simulink model "ROPOD_Control_SIM"  (R2017b)
settings: Solver=VariableStepAuto  StartTime=0.0  StopTime=inf  RelTol=1e-3
values from neighbouring files (symbols this model uses):
  AgentNumber = 1    [init_model.m]
  FFtheta_intia = 0    [init_model.m]
  FFxy_mass = 0*80    (= 0)    [init_model.m]
  flock_FFtheta_friction = 50    [init_model.m]
  flock_FFxy_friction = 100    [init_model.m]
  I_fhz_ddelta_cntr = 0    [init_model.m]
  I_fhz_dtheta_cntr = 0.3    [init_model.m]
  I_fhz_dtheta_flock_cntr = 0.1    [init_model.m]
  I_fhz_dvarphi_cntr = 0    [init_model.m]
  I_fhz_dxdy_cntr = 0.25    [init_model.m]
  I_fhz_dxdy_flock_cntr = 0.1    [init_model.m]
  K_gain_ddelta_cntr = 0.1    [init_model.m]
  K_gain_dtheta_cntr = 150    [init_model.m]
  K_gain_dtheta_flock_cntr = 100    [init_model.m]
  K_gain_dvarphi_cntr = 0.05    [init_model.m]
  K_gain_dxdy_cntr = 200    [init_model.m]
  K_gain_dxdy_flock_cntr = 200    [init_model.m]
  LL_wp_fhz_ddelta_cntr = 2    [init_model.m]
  LL_wp_fhz_dtheta_cntr = 20    [init_model.m]
  LL_wp_fhz_dtheta_flock_cntr = 20    [init_model.m]
  LL_wp_fhz_dvarphi_cntr = 10    [init_model.m]
  LL_wp_fhz_dxdy_cntr = 20    [init_model.m]
  LL_wp_fhz_dxdy_flock_cntr = 20    [init_model.m]
  LL_wz_fhz_ddelta_cntr = 2    [init_model.m]
  LL_wz_fhz_dtheta_cntr = 20    [init_model.m]
  LL_wz_fhz_dtheta_flock_cntr = 20    [init_model.m]
  LL_wz_fhz_dvarphi_cntr = 2    [init_model.m]
  LL_wz_fhz_dxdy_cntr = 20    [init_model.m]
  LL_wz_fhz_dxdy_flock_cntr = 20    [init_model.m]
  LPF_fhz_ddelta_cntr = 50    [init_model.m]
  LPF_fhz_ddelta_meas = 50    [init_model.m]
  LPF_fhz_dtheta_cntr = 100    [init_model.m]
  LPF_fhz_dtheta_flock_cntr = 40    [init_model.m]
  LPF_fhz_dvarphi_cntr = 50    [init_model.m]
  LPF_fhz_dvarphi_meas = 50    [init_model.m]
  LPF_fhz_dxdy_cntr = 100    [init_model.m]
  LPF_fhz_dxdy_flock_cntr = 40    [init_model.m]
  max_flock_acc_theta = 0.5    [init_model.m]
  max_flock_acc_xy = 0.5    [init_model.m]
  max_flock_vel_theta = 1.0    (= 1)    [init_model.m]
  max_flock_vel_xy = 1.0    (= 1)    [init_model.m]
  max_hw_tau = 7.0    (= 7)    [init_model.m]
  max_ropod_acc_theta = 1.6    [init_model.m]
  max_ropod_acc_xy = 2.0    (= 2)    [init_model.m]
  max_ropod_sw_force = 500    [init_model.m]
  max_ropod_sw_tau = 250    [init_model.m]
  max_ropod_vel_theta = 1.6    [init_model.m]
  max_ropod_vel_xy = 2.0    (= 2)    [init_model.m]
  max_sw_current = 10    [init_model.m]
  Nagents = 2    [init_model.m]
  Nwheels = 4    [Jqwl_numeric_function.m]    (also in S_matrix.m; extract_kinmodel_parameters.m; init_model.m; tau_optimal_dist_vec_fun.m)
  pivot_offs_sws = [0.0243    0.4689    0.3384    5.9050]    [init_model.m]
  ropod_kinmodel_pv = struct2array(ropod_kinmodel_param)    [set_ropod_KinModparams.m]
  ropod_position_inflock = [-1 0 3.1416]    [init_model.m]
  SW_COM1_ENABLE1 = hex2dec('0001')    [init_model.m]
  SW_COM1_ENABLE2 = hex2dec('0002')    [init_model.m]
  SW_COM1_MODE_TORQUE = bitshift(hex2dec('0000'),2)    [init_model.m]
  SW_COM1_MODE_VELOCITY = bitshift(hex2dec('0002'),2)    [init_model.m]
  SW_COM1_USE_TS = hex2dec('8000')    [init_model.m]
  sw_tau_2_current = 1/motor_physical_parameters.torqueconstant.value    [init_model.m]
  Tinit = 2    [init_model.m]
  Ts = 0.001    [init_model.m]
  Ts_MPC = 0.01    [init_model.m]
  Tsflck = 0.01    [init_model.m]
undefined symbols (not defined in the file or in its folder): acc_limit, accmax, b_cx, b_cy, b_rx, bus_size, comp_enable, Desired, DiscIntNeverNeededParam, Fcgain, gdis, k_cx, k_cy, live_tuning, m_robot, Nominal, Nominal_x, Nominal_y, offsets, portwidth, sizes, types, vel_limit, vmax1, vmax2
libraries: simulink x90, cstblocks x66, dspsigops x12, dspnetwork x4
(part 8 of 8)

== matlab function ROPOD_Control_SIM/RopodTorqueDistribution/wheel flip compensation/MATLAB Function2 ==
  data: tl input; tl_out output; tr input; ropod_kinmodel_param_vec input size=18; tr_out output; kmax input; sc output; Fthr input; tau_max input
function [tl_out,tr_out, sc] = fcn(tl, tr, ropod_kinmodel_param_vec, kmax, Fthr, tau_max)

[  rW1_1,rW1_2,rW1_3,rW1_4,rW2_1,rW2_2,rW2_3,rW2_4,...
    s_w,...
    d_w, ...
    CW1_1,CW1_2,CW1_3,CW1_4,CW2_1,CW2_2,CW2_3,CW2_4 ...
    ]= extract_kinmodel_parameters(ropod_kinmodel_param_vec);

Fxi = (tl/rW1_1+tr/rW1_2);
Fyi = (tr/rW1_2-tl/rW1_1)*(d_w/(2*s_w));
theta = atan2(Fyi,Fxi);

Fsize = abs(Fyi);
if Fsize> Fthr
   sc = (1+(kmax-1)*abs( sin(theta)) );
else
    sc = 1;
end

avg_t = (tr+tl)/2;
diff_t = (tr-tl)/2;
tl_out = avg_t-sc*diff_t;
tr_out = avg_t+sc*diff_t;

if(abs(tl_out)>tau_max && abs(tl_out)>abs(tr_out))
    sc = tau_max/abs(tl_out);
    tl_out = sc*tl_out;
    tr_out = sc*tr_out;
end

if(abs(tr_out)>tau_max && abs(tr_out)>abs(tl_out))
    sc = tau_max/abs(tr_out);
    tl_out = sc*tl_out;
    tr_out = sc*tr_out;
end

== matlab function ROPOD_Control_SIM/RopodTorqueDistribution/wheel flip compensation/MATLAB Function3 ==
  data: tl input; tl_out output; tr input; ropod_kinmodel_param_vec input size=18; tr_out output; kmax input; sc output; Fthr input; tau_max input
function [tl_out,tr_out, sc] = fcn(tl, tr, ropod_kinmodel_param_vec, kmax, Fthr, tau_max)

[  rW1_1,rW1_2,rW1_3,rW1_4,rW2_1,rW2_2,rW2_3,rW2_4,...
    s_w,...
    d_w, ...
    CW1_1,CW1_2,CW1_3,CW1_4,CW2_1,CW2_2,CW2_3,CW2_4 ...
    ]= extract_kinmodel_parameters(ropod_kinmodel_param_vec);

Fxi = (tl/rW1_1+tr/rW1_2);
Fyi = (tr/rW1_2-tl/rW1_1)*(d_w/(2*s_w));
theta = atan2(Fyi,Fxi);

Fsize = abs(Fyi);
if Fsize> Fthr
   sc = (1+(kmax-1)*abs( sin(theta)) );
else
    sc = 1;
end

avg_t = (tr+tl)/2;
diff_t = (tr-tl)/2;
tl_out = avg_t-sc*diff_t;
tr_out = avg_t+sc*diff_t;

if(abs(tl_out)>tau_max && abs(tl_out)>abs(tr_out))
    sc = tau_max/abs(tl_out);
    tl_out = sc*tl_out;
    tr_out = sc*tr_out;
end

if(abs(tr_out)>tau_max && abs(tr_out)>abs(tl_out))
    sc = tau_max/abs(tr_out);
    tl_out = sc*tl_out;
    tr_out = sc*tr_out;
end

== matlab function ROPOD_Control_SIM/RopodTorqueDistribution/Torque distribution using pseudoinverse/platform_forces_2_tau_dist_optimal_pseudo_inverse ==
  data: GtSl input; taubody input; ena_w input; varphi_tau output; tau_max input; taubody_sc output
function [varphi_tau, taubody_sc]   = Ttaud_optimal_vec( GtSl, taubody, ena_w , tau_max)
%#codegen

Nwheels = 4;

% Optimization
M = eye(2*Nwheels);
for idx = 1:Nwheels
    M(2*(idx-1)+1,2*(idx-1)+1) = ena_w(idx);
    M(2*(idx-1)+2,2*(idx-1)+2) = ena_w(idx);
end
GtM = GtSl*M;

varphi_tau_int = pinv(GtM)*taubody;
varphi_tau_int_max = max(abs(varphi_tau_int));
 

if(varphi_tau_int_max > tau_max)
    taubody_sc = tau_max/varphi_tau_int_max;
else
    taubody_sc = 1.0;
end

varphi_tau = taubody_sc*varphi_tau_int;

end

== matlab function ROPOD_Control_SIM/FlockController/MATLAB Function ==
  data: w_agents_setp input; agents_setp output; d_agents_setp input
function agents_setp = fcn(w_agents_setp, d_agents_setp)

% 3 from three degrees of freedom
% 2 from 1 wrench command +1 velocity command
Nagents = (length(w_agents_setp)/3)+1;
agents_setp_ = zeros(1,2*3*(Nagents-1));

for i_agnt = 1:Nagents-1
    agents_setp_(2*3*(i_agnt-1)+1:2*3*(i_agnt-1)+3) = w_agents_setp(3*(i_agnt-1)+1:3*(i_agnt-1)+3);
    agents_setp_(2*3*(i_agnt-1)+4:2*3*(i_agnt-1)+6) = d_agents_setp(3*(i_agnt-1)+1:3*(i_agnt-1)+3);
end

agents_setp = agents_setp_;

== matlab function ROPOD_Control_SIM/RopodTorqueDistribution/wheel flip compensation/MATLAB Function4 ==
  data: tl input; tl_out output; tr input; ropod_kinmodel_param_vec input size=18; tr_out output; kmax input; sc output; Fthr input; tau_max input
function [tl_out,tr_out, sc] = fcn(tl, tr, ropod_kinmodel_param_vec, kmax, Fthr, tau_max)

[  rW1_1,rW1_2,rW1_3,rW1_4,rW2_1,rW2_2,rW2_3,rW2_4,...
    s_w,...
    d_w, ...
    CW1_1,CW1_2,CW1_3,CW1_4,CW2_1,CW2_2,CW2_3,CW2_4 ...
    ]= extract_kinmodel_parameters(ropod_kinmodel_param_vec);

Fxi = (tl/rW1_1+tr/rW1_2);
Fyi = (tr/rW1_2-tl/rW1_1)*(d_w/(2*s_w));
theta = atan2(Fyi,Fxi);

Fsize = abs(Fyi);
if Fsize> Fthr
   sc = (1+(kmax-1)*abs( sin(theta)) );
else
    sc = 1;
end

avg_t = (tr+tl)/2;
diff_t = (tr-tl)/2;
tl_out = avg_t-sc*diff_t;
tr_out = avg_t+sc*diff_t;

if(abs(tl_out)>tau_max && abs(tl_out)>abs(tr_out))
    sc = tau_max/abs(tl_out);
    tl_out = sc*tl_out;
    tr_out = sc*tr_out;
end

if(abs(tr_out)>tau_max && abs(tr_out)>abs(tl_out))
    sc = tau_max/abs(tr_out);
    tl_out = sc*tl_out;
    tr_out = sc*tr_out;
end

== matlab function ROPOD_Control_SIM/RopodProcessWheelSensorData/Odometry and Measurement model 4SW/Jqwl_numeric ==
  data: ropod_kinmodel_param_vec input; v output; delta input; dvarphi input; ena_w input
function v = Jqwl_numeric_wrapper(ropod_kinmodel_param_vec,  delta, dvarphi, ena_w)

v = Jqwl_numeric_function(ropod_kinmodel_param_vec, delta, dvarphi, ena_w);

end

== matlab function ROPOD_Control_SIM/RopodProcessWheelSensorData/Odometry and Measurement model 4SW/pos_rot_matrix ==
  data: dqr_loc input; theta_odom input; dqr_glb output
function dqr_glb   = zrot(dqr_loc, theta_odom)
%ROPOD_JACOBIAN Summary of this function goes here
%   Detailed explanation goes here


dqr_glb = [  cos(theta_odom) -sin(theta_odom) 0; 
            sin(theta_odom)  cos(theta_odom) 0;
                    0             0  1]*dqr_loc;
end

== matlab function ROPOD_Control_SIM/Subsystem1/Compliant control/Impedance/Impedance control ==
  data: x0i input; y0i input; theta0i input; q1 input size=[2,1]; q2 input size=[2,1]; q3 input size=[2,1]; Fext input; F output; Desired parameter; Nominal parameter; vmax1 parameter; vmax2 parameter; vel_limit parameter; params_xy input; live_tuning parameter
function F = fcn(x0i,y0i,theta0i,q1,q2,q3,Fext,Desired,Nominal,vmax1,vmax2,vel_limit,params_xy, live_tuning)

q = [q1(1);q2(1);q3(1)]; %Position of system
qd = [q1(2);q2(2);q3(2)]; %Velocity of system

q0 = [x0i(1); y0i(1); theta0i(1)]; %Position reference, not really used
q0d = [x0i(2); y0i(2); theta0i(2)]; %Velocity reference, not really used
q0dd = [x0i(3); y0i(3); theta0i(3)]; %Acceleration referece, not really used

Md = Desired.mass; 
Dd = Desired.damping; 
Kd = Desired.stiffness;

Fdd = Desired.Fd; 
Fdn = Nominal.Fd;

if live_tuning && sum(params_xy) > 0
    Md(1:2) = [params_xy(1); params_xy(1)];
    Dd(1:2) = [params_xy(2); params_xy(2)];
    Fdd(1:2) = [params_xy(3); params_xy(3)];
    vel_limit = params_xy(4);
end

e = q-q0; %Position error
ed = qd-q0d; %Velocity error
m = Nominal.mass;
d = Nominal.damping;

vector = [1;1;0.2];

totv = sqrt(sum((qd.*vector).^2)); %Total velocity of system
totve = sqrt(sum((ed.*vector).^2)); %Total velocity error


if vel_limit
    
    t.magnitude = 0.5;
    t.offset = 0.5;
    t.freq = ((vmax2-vmax1)^(-1)*2*pi)/2;
    
    if totv < vmax1
        scaling = 1;
    elseif totv >= vmax1 && totv < vmax2
        scaling = t.offset + t.magnitude*cos(t.freq*(totv-vmax1));
    else
        scaling = 0;
    end
    
    Md = m + (Md-m)*scaling;
    Dd = d + (Dd-d)*scaling;
    Fdd = Fdn + (Fdd-Fdn)*scaling;
    Kd = 0 + (Kd-0)*scaling;
    
end

if totv == 0
    totv = 1;
end
if totve == 0
    totve = 1;
end

Fricn = abs(qd.*vector./totv).*tanh(40.*qd.*vector).*Fdn;
Fricd = abs(ed.*vector./totve).*tanh(40.*ed.*vector).*Fdd;

% F = d*yd - Fext + m*y0dd + Fdn*tanh(200*yd) - (m*(Kd*ey - Fext - Dd*y0d + Dd*yd + Fdd*tanh(200*eyd)))/Md; %Custom system with damp and fric
F = d.*qd - Fext + m.*q0dd + Fricn - (m.*(Kd.*e - Fext - Dd.*q0d + Dd.*qd + Fricd))./Md; %Custom system with damp and fric
% F(3) = 0;
% totv = sqrt(qd(1)^2+qd(2)^2);
% totve = sqrt(ed(1)^2+ed(2)^2);
% totv = sqrt(sum(qd.^2));
% totve = sqrt(sum(ed.^2));
% Fricv = Fdn*tanh(40*totv);
% Frice = Fdd*tanh(40*totve);

% if totv == 0
%     totv = 1;
% end
% if totve == 0
%     totve = 1;
% end

% F(1:2,1) = F(1:2,1) + Fricn - m*Fricd/Md;
% F(1:2,1) = F(1:2,1) + qd.*(Fricv/totv) - m.*qd.*(Frice/totve)/Md;
% F(3,1) = do*q3(2) - Fext(3) + mo*theta0i(3) + Fdno*tanh(40*q3(2)) - (mo*(Kdo*eo - Fext(3) - Ddo*theta0i(2) + Ddo*q3(2) + Fddo*tanh(40*edo)))/Mdo;

== matlab function ROPOD_Control_SIM/Subsystem2/ZMPC_1d_x/MATLAB Function ==
  data: m_r input; F output; b_r input; b_c input; k_c input; Fd_max input; Fd_min input; l_max input; l_min input; Fr_max input; Fr_min input; Ts_MPC input; W output; c output; H output; A output; rho output; update input
function [F, W, c, H, A, rho] = generateMPCmatrices_wrapper(m_r,  b_r, b_c, k_c, Fd_max, Fd_min, l_max, l_min, Fr_max, Fr_min, Ts_MPC, update)

[F, W, c, H, A, rho] = generateMPCmatrices(m_r,  b_r, b_c, k_c, Fd_max, Fd_min, l_max, l_min, Fr_max, Fr_min, Ts_MPC, update);

== matlab function ROPOD_Control_SIM/Subsystem2/ZMPC_1d_x/Zone MPC ==
  data: epsilon output; u_mpc output size=1; xk input size=4; F input; W input; c input; H input; A input; rho input; exitflag output
function [epsilon, u_mpc, exitflag] = Zone_MPC_wrapper(xk, F, W, c, H, A, rho)

[epsilon, u_mpc, exitflag] = Zone_MPC(xk, F, W, c, H, A, rho);

end

== matlab function ROPOD_Control_SIM/Subsystem2/ZMPC_1d_y/MATLAB Function ==
  data: m_r input; F output; b_r input; b_c input; k_c input; Fd_max input; Fd_min input; l_max input; l_min input; Fr_max input; Fr_min input; Ts_MPC input; W output; c output; H output; A output; rho output; update input
function [F, W, c, H, A, rho] = generateMPCmatrices_wrapper(m_r,  b_r, b_c, k_c, Fd_max, Fd_min, l_max, l_min, Fr_max, Fr_min, Ts_MPC, update)

[F, W, c, H, A, rho] = generateMPCmatrices(m_r,  b_r, b_c, k_c, Fd_max, Fd_min, l_max, l_min, Fr_max, Fr_min, Ts_MPC, update);

== matlab function ROPOD_Control_SIM/Subsystem2/ZMPC_1d_y/Zone MPC ==
  data: epsilon output; u_mpc output size=1; xk input size=4; F input; W input; c input; H input; A input; rho input; exitflag output
function [epsilon, u_mpc, exitflag] = Zone_MPC_wrapper(xk, F, W, c, H, A, rho)

[epsilon, u_mpc, exitflag] = Zone_MPC(xk, F, W, c, H, A, rho);

end

== matlab function ROPOD_Control_SIM/Subsystem2/Bumper_system/Force_per_sensor ==
  data: s_data_Xp input; Force_Torque output; s_data_Xm input; s_data_Yp input; s_data_Ym input; k_cx input; b_cx input; k_cy input; b_cy input
function Force_Torque  = Sensor_data(s_data_Xp, s_data_Xm, s_data_Yp, s_data_Ym, k_cx, b_cx, k_cy, b_cy)
Force_Xp = zeros(1,4);
Force_Xm = zeros(1,4);
Force_Yp = zeros(1,4);
Force_Ym = zeros(1,4);
Torque_Xp = zeros(1,4);
Torque_Xm = zeros(1,4);
Torque_Yp = zeros(1,4);
Torque_Ym = zeros(1,4);
sd = 0.164; % sensor distance [m]


Force_Xp(1) = k_cx*s_data_Xp(1) + b_cx*s_data_Xp(5);
Force_Xp(2) = k_cx*s_data_Xp(2) + b_cx*s_data_Xp(6);
Force_Xp(3) = k_cx*s_data_Xp(3) + b_cx*s_data_Xp(7);
Force_Xp(4) = k_cx*s_data_Xp(4) + b_cx*s_data_Xp(8);

Torque_Xp(1) = Force_Xp(1)*1.5*sd;
Torque_Xp(2) = Force_Xp(2)*sd;
Torque_Xp(3) = Force_Xp(3)*-sd;
Torque_Xp(4) = Force_Xp(4)*-1.5*sd;

Force_Xm(1) = k_cx*s_data_Xm(1) + b_cx*s_data_Xm(5);
Force_Xm(2) = k_cx*s_data_Xm(2) + b_cx*s_data_Xm(6);
Force_Xm(3) = k_cx*s_data_Xm(3) + b_cx*s_data_Xm(7);
Force_Xm(4) = k_cx*s_data_Xm(4) + b_cx*s_data_Xm(8);

Torque_Xm(1) = Force_Xm(1)*1.5*sd;
Torque_Xm(2) = Force_Xm(2)*sd;
Torque_Xm(3) = Force_Xm(3)*-sd;
Torque_Xm(4) = Force_Xm(4)*-1.5*sd;

Force_Yp(1) = k_cy*s_data_Yp(1) + b_cy*s_data_Yp(5);
Force_Yp(2) = k_cy*s_data_Yp(2) + b_cy*s_data_Yp(6);
Force_Yp(3) = k_cy*s_data_Yp(3) + b_cy*s_data_Yp(7);
Force_Yp(4) = k_cy*s_data_Yp(4) + b_cy*s_data_Yp(8);

Torque_Yp(1) = Force_Yp(1)*1.5*sd;
Torque_Yp(2) = Force_Yp(2)*sd;
Torque_Yp(3) = Force_Yp(3)*-sd;
Torque_Yp(4) = Force_Yp(4)*-1.5*sd;

Force_Ym(1) = k_cy*s_data_Ym(1) + b_cy*s_data_Ym(5);
Force_Ym(2) = k_cy*s_data_Ym(2) + b_cy*s_data_Ym(6);
Force_Ym(3) = k_cy*s_data_Ym(3) + b_cy*s_data_Ym(7);
Force_Ym(4) = k_cy*s_data_Ym(4) + b_cy*s_data_Ym(8);

Torque_Ym(1) = Force_Ym(1)*1.5*sd;
Torque_Ym(2) = Force_Ym(2)*sd;
Torque_Ym(3) = Force_Ym(3)*-sd;
Torque_Ym(4) = Force_Ym(4)*-1.5*sd;

Force_Torque = [sum(Force_Xp); sum(Torque_Xp); sum(Force_Yp); sum(Torque_Yp); sum(Force_Xm); sum(Torque_Xm); sum(Force_Ym); sum(Torque_Ym)]

end

== matlab function ROPOD_Control_SIM/Subsystem2/Bumper_system/cal/Calibration1 ==
  data: angle input; cal_angle output; sample input; i output; data input; data_out output
function [cal_angle, i, data_out]= fcn(angle,sample,data)
cal_start_sample = 5000;
cal_end_sample = 6000;

if sample > cal_start_sample && sample <= cal_end_sample
    data_out = data+angle; 
    cal_angle = angle;
else
    correction = data/(cal_end_sample - cal_start_sample);
    cal_angle = angle-correction;
    data_out = data;
end

i = sample+1;

== matlab function ROPOD_Control_SIM/Subsystem2/Bumper_system/cal1/Calibration1 ==
  data: cal_done output; angle input; cal_angle output; sample input; i output; data input; data_out output
function [cal_done, cal_angle, i, data_out]= fcn(angle,sample,data)
cal_start_sample = 5000;
cal_end_sample = 6000;

if sample > cal_start_sample && sample <= cal_end_sample
    data_out = data+angle; 
    cal_angle = angle;
else
    correction = data/(cal_end_sample - cal_start_sample);
    cal_angle = angle-correction;
    data_out = data;
end

if sample > cal_end_sample
    cal_done = 1;
else
    cal_done = 0;
end


i = sample+1;

== matlab function ROPOD_Control_SIM/Subsystem2/Bumper_system/cal2/Calibration1 ==
  data: angle input; cal_angle output; sample input; i output; data input; data_out output
function [cal_angle, i, data_out]= fcn(angle,sample,data)
cal_start_sample = 5000;
cal_end_sample = 6000;

if sample > cal_start_sample && sample <= cal_end_sample
    data_out = data+angle; 
    cal_angle = angle;
else
    correction = data/(cal_end_sample - cal_start_sample);
    cal_angle = angle-correction;
    data_out = data;
end

i = sample+1;

== matlab function ROPOD_Control_SIM/Subsystem2/Bumper_system/cal3/Calibration1 ==
  data: angle input; cal_angle output; sample input; i output; data input; data_out output
function [cal_angle, i, data_out]= fcn(angle,sample,data)
cal_start_sample = 5000;
cal_end_sample = 6000;

if sample > cal_start_sample && sample <= cal_end_sample
    data_out = data+angle; 
    cal_angle = angle;
else
    correction = data/(cal_end_sample - cal_start_sample);
    cal_angle = angle-correction;
    data_out = data;
end

i = sample+1;

== matlab function ROPOD_Control_SIM/Subsystem2/Bumper_system/cal4/Calibration1 ==
  data: angle input; cal_angle output; sample input; i output; data input; data_out output
function [cal_angle, i, data_out]= fcn(angle,sample,data)
cal_start_sample = 5000;
cal_end_sample = 6000;

if sample > cal_start_sample && sample <= cal_end_sample
    data_out = data+angle; 
    cal_angle = angle;
else
    correction = data/(cal_end_sample - cal_start_sample);
    cal_angle = angle-correction;
    data_out = data;
end

i = sample+1;

== matlab function ROPOD_Control_SIM/Subsystem2/Bumper_system/cal5/Calibration1 ==
  data: angle input; cal_angle output; sample input; i output; data input; data_out output
function [cal_angle, i, data_out]= fcn(angle,sample,data)
cal_start_sample = 5000;
cal_end_sample = 6000;

if sample > cal_start_sample && sample <= cal_end_sample
    data_out = data+angle; 
    cal_angle = angle;
else
    correction = data/(cal_end_sample - cal_start_sample);
    cal_angle = angle-correction;
    data_out = data;
end

i = sample+1;

== matlab function ROPOD_Control_SIM/Subsystem2/Bumper_system/cal6/Calibration1 ==
  data: angle input; cal_angle output; sample input; i output; data input; data_out output
function [cal_angle, i, data_out]= fcn(angle,sample,data)
cal_start_sample = 5000;
cal_end_sample = 6000;

if sample > cal_start_sample && sample <= cal_end_sample
    data_out = data+angle; 
    cal_angle = angle;
else
    correction = data/(cal_end_sample - cal_start_sample);
    cal_angle = angle-correction;
    data_out = data;
end

i = sample+1;

== matlab function ROPOD_Control_SIM/Subsystem2/Bumper_system/cal7/Calibration1 ==
  data: angle input; cal_angle output; sample input; i output; data input; data_out output
function [cal_angle, i, data_out]= fcn(angle,sample,data)
cal_start_sample = 5000;
cal_end_sample = 6000;

if sample > cal_start_sample && sample <= cal_end_sample
    data_out = data+angle; 
    cal_angle = angle;
else
    correction = data/(cal_end_sample - cal_start_sample);
    cal_angle = angle-correction;
    data_out = data;
end

i = sample+1;

== matlab function ROPOD_Control_SIM/Subsystem2/Bumper_system/speed deflection angle calculation X- ==
  data: s_data input; Total_deflection output; Total_speed output
function [Total_deflection, Total_speed] = Sensor_data(s_data)
% s_data is the sensor data
% s_data(1:4) = deflection in m
% s_data(5:8) = speed in m/s


dx = s_data(1:4); %deflection in m
dx_dot = s_data(5:8); %speed in m/s



% Deflection and speed in x direction
Total_deflection = sum(dx);
Total_speed = sum(dx_dot);



end

== matlab function ROPOD_Control_SIM/Subsystem2/Bumper_system/speed deflection angle calculation X+ ==
  data: s_data input; Total_deflection output; Total_speed output
function [Total_deflection, Total_speed] = Sensor_data(s_data)
% s_data is the sensor data
% s_data(1:4) = deflection in m
% s_data(5:8) = speed in m/s


dx = s_data(1:4); %deflection in m
dx_dot = s_data(5:8); %speed in m/s



% Deflection and speed in x direction
Total_deflection = sum(dx);
Total_speed = sum(dx_dot);



end

== matlab function ROPOD_Control_SIM/Subsystem2/Bumper_system/speed deflection angle calculation Y+ ==
  data: s_data input; Total_deflection output; Total_speed output
function [Total_deflection, Total_speed] = Sensor_data(s_data)
% s_data is the sensor data
% s_data(1:4) = deflection in m
% s_data(5:8) = speed in m/s


dx = s_data(1:4); %deflection in m
dx_dot = s_data(5:8); %speed in m/s



% Deflection and speed in x direction
Total_deflection = sum(dx);
Total_speed = sum(dx_dot);



end

== matlab function ROPOD_Control_SIM/Subsystem2/Bumper_system/speed deflection angle calculation Y- ==
  data: s_data input; Total_deflection output; Total_speed output
function [Total_deflection, Total_speed] = Sensor_data(s_data)
% s_data is the sensor data
% s_data(1:4) = deflection in m
% s_data(5:8) = speed in m/s


dx = s_data(1:4); %deflection in m
dx_dot = s_data(5:8); %speed in m/s



% Deflection and speed in x direction
Total_deflection = sum(dx);
Total_speed = sum(dx_dot);



end

== matlab function ROPOD_Control_SIM/ropod_coordination_state_machine ==
  data: ropod_cntr_state output; initialize input; ropod_cntr_mode output; ropod_enable input; flock_mode input; enable_zmpc_fx input; enable_zmpc_fy input; reenable_vel_cntr input; bpr_calibration input; select_w_x output; select_w_y output; select_w_rz output; select_dq output
function [ropod_cntr_state, ropod_cntr_mode, select_w_x, select_w_y, select_w_rz, select_dq] = ropod_coordination_state_machine(initialize, ropod_enable, flock_mode, enable_zmpc_fx, enable_zmpc_fy, reenable_vel_cntr, bpr_calibration)

persistent control_state;

if isempty(control_state)
    control_state = 1;
end

VEL_CONTROL_XYT = 1;
VEL_CONTROL_XT_ZMPC_Y = 2;
ZMPC_XY_NOCNTR_T = 3;
FLOCK_CNTR = 4;

if ropod_enable
    if initialize
        ropod_cntr_mode = 2;
    else
        ropod_cntr_mode = 1;
    end
    
else
    ropod_cntr_mode = 0;
end

if bpr_calibration == 0
    % Wait for bumper calibration
    ropod_cntr_mode = 0;
    control_state = VEL_CONTROL_XYT;
end

if flock_mode > 0
    % Ignore bumper
    control_state = FLOCK_CNTR;
end
    
ropod_cntr_state = control_state;
%% Control state
switch control_state
    case VEL_CONTROL_XYT  % Velocity control x-y-theta
        select_w_x = 1;
        select_w_y = 1;
        select_w_rz = 1;
        select_dq = 1;
        
        if enable_zmpc_fy
            control_state = VEL_CONTROL_XT_ZMPC_Y;
        end
        if enable_zmpc_fx
            control_state = ZMPC_XY_NOCNTR_T;
        end
        
    case VEL_CONTROL_XT_ZMPC_Y  % Velocity control x-theta ZMPC-y
        select_w_x = 1;
        select_w_y = 3;
        select_w_rz = 1;
        select_dq = 1;
        
        if reenable_vel_cntr || enable_zmpc_fy == 0
            control_state = VEL_CONTROL_XYT;
        end
        
        if enable_zmpc_fx
            control_state = ZMPC_XY_NOCNTR_T;
        end
        
    case ZMPC_XY_NOCNTR_T  % ZMPC x-y no control on theta
        select_w_x = 3;
        select_w_y = 3;
        select_w_rz = 3;
        select_dq = 3;
        
        if reenable_vel_cntr
            control_state = VEL_CONTROL_XYT;
        end

    case FLOCK_CNTR % Flock control
        select_w_x = 2;
        select_w_y = 2;
        select_w_rz = 2;
        select_dq = 2;
        
    otherwise
        select_w_x = 1;
        select_w_y = 1;
        select_w_rz = 1;
        select_dq = 1;
        control_state = VEL_CONTROL_XYT;
end
